simulink model "HGDiff"  (R2016b)
settings: Solver=VariableStepAuto  StartTime=0.0  StopTime=10.0  RelTol=1e-3
values from neighbouring files (symbols this model uses):
  K = 100    [DiffSim.m]
libraries: dsparch4 x1
settings Model: Creator=lucac  LastModifiedBy=lucac

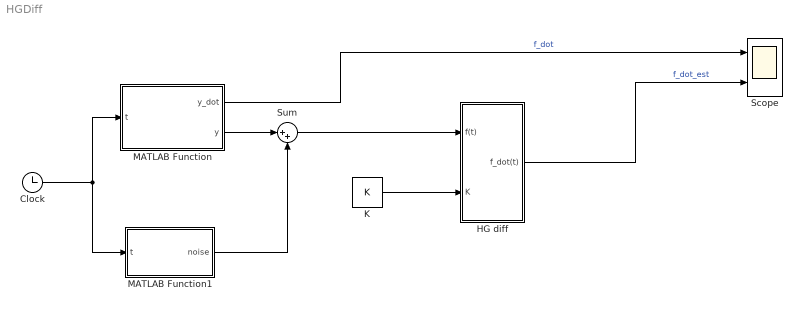
== system HGDiff ==
  Clock : Clock
  HG diff : Subsystem
  K : Constant  Value=K
  MATLAB Function : MATLAB Function  TreatAsAtomicUnit=on
  MATLAB Function1 : MATLAB Function  TreatAsAtomicUnit=on
  Scope : Scope  NumInputPorts=2
  Sum : Sum  Inputs=|++
  wires:
  Clock/1 -> MATLAB Function/1(t), MATLAB Function1/1(t)
  K/1 -> HG diff/2(K)
  HG diff/1(f_dot(t)) -> Scope/2  "f_dot_est"
  MATLAB Function/1(y_dot) -> Scope/1  "f_dot"
  MATLAB Function/2(y) -> Sum/1
  Sum/1 -> HG diff/1(f(t))
  MATLAB Function1/1(noise) -> Sum/2

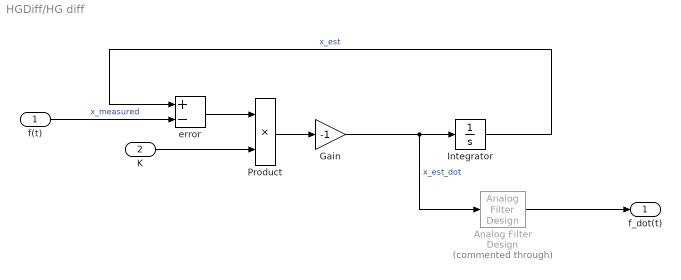
== system HGDiff/HG diff ==
  f(t) : Inport
  K : Inport  Port=2
  Analog Filter Design : dsparch4/Analog Filter Design  Commented=through  method=Butterworth  filttype=Lowpass  N=1  Wlo=20  Whi=80  Rp=2  Rs=40
  Gain : Gain  Gain=-1
  Integrator : Integrator
  Product : Product
  error : Sum  Inputs=+-
  f_dot(t) : Outport
  wires:
  f(t)/1 -> error/2  "x_measured"
  Integrator/1 -> error/1  "x_est"
  Gain/1 -> Analog Filter Design/1, Integrator/1  "x_est_dot"
  Product/1 -> Gain/1
  error/1 -> Product/1
  K/1 -> Product/2
  Analog Filter Design/1 -> f_dot(t)/1

== matlab function HGDiff/MATLAB Function1 ==
  data: t input; noise output
function noise = fcn(t)

noise = 0.001*cos(30*t);

== matlab function HGDiff/MATLAB Function ==
  data: y_dot output; t input; y output
function [y_dot, y] = fcn(t)


y_dot = 3*cos(3*t) + 2*sin(t);
y = sin(3*t) - 2*cos(t);
